simulink model "differential_equation"  (R2021a)
settings: Solver=VariableStepAuto  StartTime=0.0  StopTime=1  RelTol=1e-3
settings Model: Creator=SA  LastModifiedBy=SA

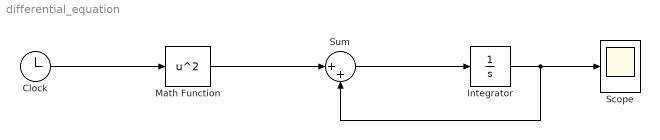
== system differential_equation ==
  Clock : Clock
  Integrator : Integrator
  Math Function : Math  Operator=square  SaturateOnIntegerOverflow=on
  Scope : Scope
  Sum : Sum  Inputs=|++
  wires:
  Clock/1 -> Math Function/1
  Math Function/1 -> Sum/1
  Sum/1 -> Integrator/1
  Integrator/1 -> Sum/2, Scope/1
